simulink model "PTControl"  (Simulink 8.7)
settings: Solver=ode45  StartTime=0.0  StopTime=inf  RelTol=1e-3
libraries: CarMaker4SL x2
(part 3 of 3)

== system PTControl/CarMaker/IPG Vehicle/PowerTrain/PTControl Example/PTControl_In/CreateBus PTC GearBoxM_In3 ==
  In : Inport
  BusCreator : BusCreator  Inputs=20
  Demux : Demux  Outputs=20
  Out : Outport
  wires:
  Demux/20 -> BusCreator/20  "PTC GearBoxM_In3 Clutch_dis i_TrqIn2Out"
  Demux/19 -> BusCreator/19  "PTC GearBoxM_In3 Clutch_dis Trq_out"
  Demux/18 -> BusCreator/18  "PTC GearBoxM_In3 Clutch_dis Trq_in"
  Demux/17 -> BusCreator/17  "PTC GearBoxM_In3 Clutch_dis rotv_out"
  Demux/16 -> BusCreator/16  "PTC GearBoxM_In3 Clutch_dis rotv_in"
  Demux/15 -> BusCreator/15  "PTC GearBoxM_In3 Clutch_dis Pos"
  Demux/14 -> BusCreator/14  "PTC GearBoxM_In3 Clutch i_TrqIn2Out"
  Demux/13 -> BusCreator/13  "PTC GearBoxM_In3 Clutch Trq_out"
  Demux/12 -> BusCreator/12  "PTC GearBoxM_In3 Clutch Trq_in"
  Demux/11 -> BusCreator/11  "PTC GearBoxM_In3 Clutch rotv_out"
  Demux/10 -> BusCreator/10  "PTC GearBoxM_In3 Clutch rotv_in"
  Demux/9 -> BusCreator/9  "PTC GearBoxM_In3 Clutch Pos"
  Demux/8 -> BusCreator/8  "PTC GearBoxM_In3 Trq_out"
  Demux/7 -> BusCreator/7  "PTC GearBoxM_In3 Trq_in"
  Demux/6 -> BusCreator/6  "PTC GearBoxM_In3 rotv_out"
  Demux/5 -> BusCreator/5  "PTC GearBoxM_In3 rotv_in"
  Demux/4 -> BusCreator/4  "PTC GearBoxM_In3 i"
  Demux/3 -> BusCreator/3  "PTC GearBoxM_In3 Trq_DriveSrc_trg"
  Demux/2 -> BusCreator/2  "PTC GearBoxM_In3 GearNo_dis"
  Demux/1 -> BusCreator/1  "PTC GearBoxM_In3 GearNo"
  BusCreator/1 -> Out/1
  In/1 -> Demux/1

== system PTControl/CarMaker/IPG Vehicle/PowerTrain/PTControl Example/PTControl_In/CreateBus PTC ISGIn ==
  In : Inport
  BusCreator : BusCreator  Inputs=9
  Demux : Demux  Outputs=9
  Out : Outport
  wires:
  Demux/9 -> BusCreator/9  "PTC ISGIn i_M2W_RR"
  Demux/8 -> BusCreator/8  "PTC ISGIn i_M2W_RL"
  Demux/7 -> BusCreator/7  "PTC ISGIn i_M2W_FR"
  Demux/6 -> BusCreator/6  "PTC ISGIn i_M2W_FL"
  Demux/5 -> BusCreator/5  "PTC ISGIn PwrElec"
  Demux/4 -> BusCreator/4  "PTC ISGIn TrqGen_max"
  Demux/3 -> BusCreator/3  "PTC ISGIn TrqMot_max"
  Demux/2 -> BusCreator/2  "PTC ISGIn Trq"
  Demux/1 -> BusCreator/1  "PTC ISGIn rotv"
  BusCreator/1 -> Out/1
  In/1 -> Demux/1

== system PTControl/CarMaker/IPG Vehicle/PowerTrain/PTControl Example/PTControl_In/CreateBus PTC MotorIn0 ==
  In : Inport
  BusCreator : BusCreator  Inputs=9
  Demux : Demux  Outputs=9
  Out : Outport
  wires:
  Demux/9 -> BusCreator/9  "PTC MotorIn0 i_M2W_RR"
  Demux/8 -> BusCreator/8  "PTC MotorIn0 i_M2W_RL"
  Demux/7 -> BusCreator/7  "PTC MotorIn0 i_M2W_FR"
  Demux/6 -> BusCreator/6  "PTC MotorIn0 i_M2W_FL"
  Demux/5 -> BusCreator/5  "PTC MotorIn0 PwrElec"
  Demux/4 -> BusCreator/4  "PTC MotorIn0 TrqGen_max"
  Demux/3 -> BusCreator/3  "PTC MotorIn0 TrqMot_max"
  Demux/2 -> BusCreator/2  "PTC MotorIn0 Trq"
  Demux/1 -> BusCreator/1  "PTC MotorIn0 rotv"
  BusCreator/1 -> Out/1
  In/1 -> Demux/1

== system PTControl/CarMaker/IPG Vehicle/PowerTrain/PTControl Example/PTControl_In/CreateBus PTC MotorIn1 ==
  In : Inport
  BusCreator : BusCreator  Inputs=9
  Demux : Demux  Outputs=9
  Out : Outport
  wires:
  Demux/9 -> BusCreator/9  "PTC MotorIn1 i_M2W_RR"
  Demux/8 -> BusCreator/8  "PTC MotorIn1 i_M2W_RL"
  Demux/7 -> BusCreator/7  "PTC MotorIn1 i_M2W_FR"
  Demux/6 -> BusCreator/6  "PTC MotorIn1 i_M2W_FL"
  Demux/5 -> BusCreator/5  "PTC MotorIn1 PwrElec"
  Demux/4 -> BusCreator/4  "PTC MotorIn1 TrqGen_max"
  Demux/3 -> BusCreator/3  "PTC MotorIn1 TrqMot_max"
  Demux/2 -> BusCreator/2  "PTC MotorIn1 Trq"
  Demux/1 -> BusCreator/1  "PTC MotorIn1 rotv"
  BusCreator/1 -> Out/1
  In/1 -> Demux/1

== system PTControl/CarMaker/IPG Vehicle/PowerTrain/PTControl Example/PTControl_In/CreateBus PTC MotorIn2 ==
  In : Inport
  BusCreator : BusCreator  Inputs=9
  Demux : Demux  Outputs=9
  Out : Outport
  wires:
  Demux/9 -> BusCreator/9  "PTC MotorIn2 i_M2W_RR"
  Demux/8 -> BusCreator/8  "PTC MotorIn2 i_M2W_RL"
  Demux/7 -> BusCreator/7  "PTC MotorIn2 i_M2W_FR"
  Demux/6 -> BusCreator/6  "PTC MotorIn2 i_M2W_FL"
  Demux/5 -> BusCreator/5  "PTC MotorIn2 PwrElec"
  Demux/4 -> BusCreator/4  "PTC MotorIn2 TrqGen_max"
  Demux/3 -> BusCreator/3  "PTC MotorIn2 TrqMot_max"
  Demux/2 -> BusCreator/2  "PTC MotorIn2 Trq"
  Demux/1 -> BusCreator/1  "PTC MotorIn2 rotv"
  BusCreator/1 -> Out/1
  In/1 -> Demux/1

== system PTControl/CarMaker/IPG Vehicle/PowerTrain/PTControl Example/PTControl_In/CreateBus PTC MotorIn3 ==
  In : Inport
  BusCreator : BusCreator  Inputs=9
  Demux : Demux  Outputs=9
  Out : Outport
  wires:
  Demux/9 -> BusCreator/9  "PTC MotorIn3 i_M2W_RR"
  Demux/8 -> BusCreator/8  "PTC MotorIn3 i_M2W_RL"
  Demux/7 -> BusCreator/7  "PTC MotorIn3 i_M2W_FR"
  Demux/6 -> BusCreator/6  "PTC MotorIn3 i_M2W_FL"
  Demux/5 -> BusCreator/5  "PTC MotorIn3 PwrElec"
  Demux/4 -> BusCreator/4  "PTC MotorIn3 TrqGen_max"
  Demux/3 -> BusCreator/3  "PTC MotorIn3 TrqMot_max"
  Demux/2 -> BusCreator/2  "PTC MotorIn3 Trq"
  Demux/1 -> BusCreator/1  "PTC MotorIn3 rotv"
  BusCreator/1 -> Out/1
  In/1 -> Demux/1

== system PTControl/CarMaker/IPG Vehicle/PowerTrain/PTControl Example/PTControl_In/CreateBus PTC PwrSupplyIn ==
  In : Inport
  BusCreator : BusCreator  Inputs=12
  Demux : Demux  Outputs=12
  Out : Outport
  wires:
  Demux/12 -> BusCreator/12  "PTC PwrSupplyIn Eta_HV1toHV2"
  Demux/11 -> BusCreator/11  "PTC PwrSupplyIn Eta_HV1toLV"
  Demux/10 -> BusCreator/10  "PTC PwrSupplyIn Pwr_HV1toHV2_max"
  Demux/9 -> BusCreator/9  "PTC PwrSupplyIn Pwr_HV1toLV_max"
  Demux/8 -> BusCreator/8  "PTC PwrSupplyIn Pwr_HV1toHV2"
  Demux/7 -> BusCreator/7  "PTC PwrSupplyIn Pwr_HV1toLV"
  Demux/6 -> BusCreator/6  "PTC PwrSupplyIn Voltage_HV2"
  Demux/5 -> BusCreator/5  "PTC PwrSupplyIn Voltage_HV1"
  Demux/4 -> BusCreator/4  "PTC PwrSupplyIn Voltage_LV"
  Demux/3 -> BusCreator/3  "PTC PwrSupplyIn Pwr_HV2"
  Demux/2 -> BusCreator/2  "PTC PwrSupplyIn Pwr_HV1"
  Demux/1 -> BusCreator/1  "PTC PwrSupplyIn Pwr_LV"
  BusCreator/1 -> Out/1
  In/1 -> Demux/1

== system PTControl/CarMaker/IPG Vehicle/PowerTrain/PTControl Example/PTControl_In/CreateBus PTC Vehicle Ctrl ==
  In : Inport
  BusCreator : BusCreator  Inputs=8
  Demux : Demux  Outputs=8
  Out : Outport
  wires:
  Demux/8 -> BusCreator/8  "PTC Velocity"
  Demux/7 -> BusCreator/7  "PTC Brake"
  Demux/6 -> BusCreator/6  "PTC Gas"
  Demux/5 -> BusCreator/5  "PTC Clutch"
  Demux/4 -> BusCreator/4  "PTC GearNoTrg"
  Demux/3 -> BusCreator/3  "PTC SelectorCtrl"
  Demux/2 -> BusCreator/2  "PTC SST"
  Demux/1 -> BusCreator/1  "PTC Key"
  BusCreator/1 -> Out/1
  In/1 -> Demux/1

== system PTControl/CarMaker/IPG Vehicle/PowerTrain/PTControl Example/PTControl_In/CreateBus PTC WheelIn ==
  In : Inport
  BusCreator : BusCreator  Inputs=4
  Demux : Demux
  Out : Outport
  wires:
  Demux/4 -> BusCreator/4  "PTC WheelIn_RR Trq_BrakeReg_trg"
  Demux/3 -> BusCreator/3  "PTC WheelIn_RL Trq_BrakeReg_trg"
  Demux/2 -> BusCreator/2  "PTC WheelIn_FR Trq_BrakeReg_trg"
  Demux/1 -> BusCreator/1  "PTC WheelIn_FL Trq_BrakeReg_trg"
  BusCreator/1 -> Out/1
  In/1 -> Demux/1

== system PTControl/CarMaker/IPG Vehicle/PowerTrain/PTControl Example/PTControl_In/CreateBus PTC_Cfg Battery ==
  In : Inport
  BusCreator : BusCreator  Inputs=8
  Demux : Demux  Outputs=8
  Out : Outport
  wires:
  Demux/8 -> BusCreator/8  "PTC_Cfg BattHV Voltage"
  Demux/7 -> BusCreator/7  "PTC_Cfg BattHV Capacity"
  Demux/6 -> BusCreator/6  "PTC_Cfg BattHV SOC_max"
  Demux/5 -> BusCreator/5  "PTC_Cfg BattHV SOC_min"
  Demux/4 -> BusCreator/4  "PTC_Cfg BattLV Voltage"
  Demux/3 -> BusCreator/3  "PTC_Cfg BattLV Capacity"
  Demux/2 -> BusCreator/2  "PTC_Cfg BattLV SOC_max"
  Demux/1 -> BusCreator/1  "PTC_Cfg BattLV SOC_min"
  BusCreator/1 -> Out/1
  In/1 -> Demux/1

== system PTControl/CarMaker/IPG Vehicle/PowerTrain/PTControl Example/PTControl_In/CreateBus PTC_Cfg Engine ==
  In : Inport
  BusCreator : BusCreator  Inputs=4
  Demux : Demux
  Out : Outport
  wires:
  Demux/4 -> BusCreator/4  "PTC_Cfg Engine rotv_opt"
  Demux/3 -> BusCreator/3  "PTC_Cfg Engine rotv_idle"
  Demux/2 -> BusCreator/2  "PTC_Cfg Engine rotv_max"
  Demux/1 -> BusCreator/1  "PTC_Cfg Engine Fuel_l2kWh"
  BusCreator/1 -> Out/1
  In/1 -> Demux/1

== system PTControl/CarMaker/IPG Vehicle/PowerTrain/PTControl Example/PTControl_In/CreateBus PTC_Cfg GearBox ==
  In : Inport
  BusCreator : BusCreator  Inputs=38
  Demux : Demux  Outputs=38
  Out : Outport
  wires:
  Demux/38 -> BusCreator/38  "PTC_Cfg GearBox iBGear16"
  Demux/37 -> BusCreator/37  "PTC_Cfg GearBox iBGear15"
  Demux/36 -> BusCreator/36  "PTC_Cfg GearBox iBGear14"
  Demux/35 -> BusCreator/35  "PTC_Cfg GearBox iBGear13"
  Demux/34 -> BusCreator/34  "PTC_Cfg GearBox iBGear12"
  Demux/33 -> BusCreator/33  "PTC_Cfg GearBox iBGear11"
  Demux/32 -> BusCreator/32  "PTC_Cfg GearBox iBGear10"
  Demux/31 -> BusCreator/31  "PTC_Cfg GearBox iBGear9"
  Demux/30 -> BusCreator/30  "PTC_Cfg GearBox iBGear8"
  Demux/29 -> BusCreator/29  "PTC_Cfg GearBox iBGear7"
  Demux/28 -> BusCreator/28  "PTC_Cfg GearBox iBGear6"
  Demux/27 -> BusCreator/27  "PTC_Cfg GearBox iBGear5"
  Demux/26 -> BusCreator/26  "PTC_Cfg GearBox iBGear4"
  Demux/25 -> BusCreator/25  "PTC_Cfg GearBox iBGear3"
  Demux/24 -> BusCreator/24  "PTC_Cfg GearBox iBGear2"
  Demux/23 -> BusCreator/23  "PTC_Cfg GearBox iBGear1"
  Demux/22 -> BusCreator/22  "PTC_Cfg GearBox iBGear0"
  Demux/21 -> BusCreator/21  "PTC_Cfg GearBox nBGears"
  Demux/20 -> BusCreator/20  "PTC_Cfg GearBox iFGear16"
  Demux/19 -> BusCreator/19  "PTC_Cfg GearBox iFGear15"
  Demux/18 -> BusCreator/18  "PTC_Cfg GearBox iFGear14"
  Demux/17 -> BusCreator/17  "PTC_Cfg GearBox iFGear13"
  Demux/16 -> BusCreator/16  "PTC_Cfg GearBox iFGear12"
  Demux/15 -> BusCreator/15  "PTC_Cfg GearBox iFGear11"
  Demux/14 -> BusCreator/14  "PTC_Cfg GearBox iFGear10"
  Demux/13 -> BusCreator/13  "PTC_Cfg GearBox iFGear9"
  Demux/12 -> BusCreator/12  "PTC_Cfg GearBox iFGear8"
  Demux/11 -> BusCreator/11  "PTC_Cfg GearBox iFGear7"
  Demux/10 -> BusCreator/10  "PTC_Cfg GearBox iFGear6"
  Demux/9 -> BusCreator/9  "PTC_Cfg GearBox iFGear5"
  Demux/8 -> BusCreator/8  "PTC_Cfg GearBox iFGear4"
  Demux/7 -> BusCreator/7  "PTC_Cfg GearBox iFGear3"
  Demux/6 -> BusCreator/6  "PTC_Cfg GearBox iFGear2"
  Demux/5 -> BusCreator/5  "PTC_Cfg GearBox iFGear1"
  Demux/4 -> BusCreator/4  "PTC_Cfg GearBox iFGear0"
  Demux/3 -> BusCreator/3  "PTC_Cfg GearBox nFGears"
  Demux/2 -> BusCreator/2  "PTC_Cfg GearBox ClKind"
  Demux/1 -> BusCreator/1  "PTC_Cfg GearBox GBKind"
  BusCreator/1 -> Out/1
  In/1 -> Demux/1

== system PTControl/CarMaker/IPG Vehicle/PowerTrain/PTControl Example/PTControl_In/CreateBus PTC_Cfg GearBoxM0 ==
  In : Inport
  BusCreator : BusCreator  Inputs=38
  Demux : Demux  Outputs=38
  Out : Outport
  wires:
  Demux/38 -> BusCreator/38  "PTC_Cfg GearBoxM0 iBGear16"
  Demux/37 -> BusCreator/37  "PTC_Cfg GearBoxM0 iBGear15"
  Demux/36 -> BusCreator/36  "PTC_Cfg GearBoxM0 iBGear14"
  Demux/35 -> BusCreator/35  "PTC_Cfg GearBoxM0 iBGear13"
  Demux/34 -> BusCreator/34  "PTC_Cfg GearBoxM0 iBGear12"
  Demux/33 -> BusCreator/33  "PTC_Cfg GearBoxM0 iBGear11"
  Demux/32 -> BusCreator/32  "PTC_Cfg GearBoxM0 iBGear10"
  Demux/31 -> BusCreator/31  "PTC_Cfg GearBoxM0 iBGear9"
  Demux/30 -> BusCreator/30  "PTC_Cfg GearBoxM0 iBGear8"
  Demux/29 -> BusCreator/29  "PTC_Cfg GearBoxM0 iBGear7"
  Demux/28 -> BusCreator/28  "PTC_Cfg GearBoxM0 iBGear6"
  Demux/27 -> BusCreator/27  "PTC_Cfg GearBoxM0 iBGear5"
  Demux/26 -> BusCreator/26  "PTC_Cfg GearBoxM0 iBGear4"
  Demux/25 -> BusCreator/25  "PTC_Cfg GearBoxM0 iBGear3"
  Demux/24 -> BusCreator/24  "PTC_Cfg GearBoxM0 iBGear2"
  Demux/23 -> BusCreator/23  "PTC_Cfg GearBoxM0 iBGear1"
  Demux/22 -> BusCreator/22  "PTC_Cfg GearBoxM0 iBGear0"
  Demux/21 -> BusCreator/21  "PTC_Cfg GearBoxM0 nBGears"
  Demux/20 -> BusCreator/20  "PTC_Cfg GearBoxM0 iFGear16"
  Demux/19 -> BusCreator/19  "PTC_Cfg GearBoxM0 iFGear15"
  Demux/18 -> BusCreator/18  "PTC_Cfg GearBoxM0 iFGear14"
  Demux/17 -> BusCreator/17  "PTC_Cfg GearBoxM0 iFGear13"
  Demux/16 -> BusCreator/16  "PTC_Cfg GearBoxM0 iFGear12"
  Demux/15 -> BusCreator/15  "PTC_Cfg GearBoxM0 iFGear11"
  Demux/14 -> BusCreator/14  "PTC_Cfg GearBoxM0 iFGear10"
  Demux/13 -> BusCreator/13  "PTC_Cfg GearBoxM0 iFGear9"
  Demux/12 -> BusCreator/12  "PTC_Cfg GearBoxM0 iFGear8"
  Demux/11 -> BusCreator/11  "PTC_Cfg GearBoxM0 iFGear7"
  Demux/10 -> BusCreator/10  "PTC_Cfg GearBoxM0 iFGear6"
  Demux/9 -> BusCreator/9  "PTC_Cfg GearBoxM0 iFGear5"
  Demux/8 -> BusCreator/8  "PTC_Cfg GearBoxM0 iFGear4"
  Demux/7 -> BusCreator/7  "PTC_Cfg GearBoxM0 iFGear3"
  Demux/6 -> BusCreator/6  "PTC_Cfg GearBoxM0 iFGear2"
  Demux/5 -> BusCreator/5  "PTC_Cfg GearBoxM0 iFGear1"
  Demux/4 -> BusCreator/4  "PTC_Cfg GearBoxM0 iFGear0"
  Demux/3 -> BusCreator/3  "PTC_Cfg GearBoxM0 nFGears"
  Demux/2 -> BusCreator/2  "PTC_Cfg GearBoxM0 ClKind"
  Demux/1 -> BusCreator/1  "PTC_Cfg GearBoxM0 GBKind"
  BusCreator/1 -> Out/1
  In/1 -> Demux/1

== system PTControl/CarMaker/IPG Vehicle/PowerTrain/PTControl Example/PTControl_In/CreateBus PTC_Cfg GearBoxM1 ==
  In : Inport
  BusCreator : BusCreator  Inputs=38
  Demux : Demux  Outputs=38
  Out : Outport
  wires:
  Demux/38 -> BusCreator/38  "PTC_Cfg GearBoxM1 iBGear16"
  Demux/37 -> BusCreator/37  "PTC_Cfg GearBoxM1 iBGear15"
  Demux/36 -> BusCreator/36  "PTC_Cfg GearBoxM1 iBGear14"
  Demux/35 -> BusCreator/35  "PTC_Cfg GearBoxM1 iBGear13"
  Demux/34 -> BusCreator/34  "PTC_Cfg GearBoxM1 iBGear12"
  Demux/33 -> BusCreator/33  "PTC_Cfg GearBoxM1 iBGear11"
  Demux/32 -> BusCreator/32  "PTC_Cfg GearBoxM1 iBGear10"
  Demux/31 -> BusCreator/31  "PTC_Cfg GearBoxM1 iBGear9"
  Demux/30 -> BusCreator/30  "PTC_Cfg GearBoxM1 iBGear8"
  Demux/29 -> BusCreator/29  "PTC_Cfg GearBoxM1 iBGear7"
  Demux/28 -> BusCreator/28  "PTC_Cfg GearBoxM1 iBGear6"
  Demux/27 -> BusCreator/27  "PTC_Cfg GearBoxM1 iBGear5"
  Demux/26 -> BusCreator/26  "PTC_Cfg GearBoxM1 iBGear4"
  Demux/25 -> BusCreator/25  "PTC_Cfg GearBoxM1 iBGear3"
  Demux/24 -> BusCreator/24  "PTC_Cfg GearBoxM1 iBGear2"
  Demux/23 -> BusCreator/23  "PTC_Cfg GearBoxM1 iBGear1"
  Demux/22 -> BusCreator/22  "PTC_Cfg GearBoxM1 iBGear0"
  Demux/21 -> BusCreator/21  "PTC_Cfg GearBoxM1 nBGears"
  Demux/20 -> BusCreator/20  "PTC_Cfg GearBoxM1 iFGear16"
  Demux/19 -> BusCreator/19  "PTC_Cfg GearBoxM1 iFGear15"
  Demux/18 -> BusCreator/18  "PTC_Cfg GearBoxM1 iFGear14"
  Demux/17 -> BusCreator/17  "PTC_Cfg GearBoxM1 iFGear13"
  Demux/16 -> BusCreator/16  "PTC_Cfg GearBoxM1 iFGear12"
  Demux/15 -> BusCreator/15  "PTC_Cfg GearBoxM1 iFGear11"
  Demux/14 -> BusCreator/14  "PTC_Cfg GearBoxM1 iFGear10"
  Demux/13 -> BusCreator/13  "PTC_Cfg GearBoxM1 iFGear9"
  Demux/12 -> BusCreator/12  "PTC_Cfg GearBoxM1 iFGear8"
  Demux/11 -> BusCreator/11  "PTC_Cfg GearBoxM1 iFGear7"
  Demux/10 -> BusCreator/10  "PTC_Cfg GearBoxM1 iFGear6"
  Demux/9 -> BusCreator/9  "PTC_Cfg GearBoxM1 iFGear5"
  Demux/8 -> BusCreator/8  "PTC_Cfg GearBoxM1 iFGear4"
  Demux/7 -> BusCreator/7  "PTC_Cfg GearBoxM1 iFGear3"
  Demux/6 -> BusCreator/6  "PTC_Cfg GearBoxM1 iFGear2"
  Demux/5 -> BusCreator/5  "PTC_Cfg GearBoxM1 iFGear1"
  Demux/4 -> BusCreator/4  "PTC_Cfg GearBoxM1 iFGear0"
  Demux/3 -> BusCreator/3  "PTC_Cfg GearBoxM1 nFGears"
  Demux/2 -> BusCreator/2  "PTC_Cfg GearBoxM1 ClKind"
  Demux/1 -> BusCreator/1  "PTC_Cfg GearBoxM1 GBKind"
  BusCreator/1 -> Out/1
  In/1 -> Demux/1

== system PTControl/CarMaker/IPG Vehicle/PowerTrain/PTControl Example/PTControl_In/CreateBus PTC_Cfg GearBoxM2 ==
  In : Inport
  BusCreator : BusCreator  Inputs=38
  Demux : Demux  Outputs=38
  Out : Outport
  wires:
  Demux/38 -> BusCreator/38  "PTC_Cfg GearBoxM2 iBGear16"
  Demux/37 -> BusCreator/37  "PTC_Cfg GearBoxM2 iBGear15"
  Demux/36 -> BusCreator/36  "PTC_Cfg GearBoxM2 iBGear14"
  Demux/35 -> BusCreator/35  "PTC_Cfg GearBoxM2 iBGear13"
  Demux/34 -> BusCreator/34  "PTC_Cfg GearBoxM2 iBGear12"
  Demux/33 -> BusCreator/33  "PTC_Cfg GearBoxM2 iBGear11"
  Demux/32 -> BusCreator/32  "PTC_Cfg GearBoxM2 iBGear10"
  Demux/31 -> BusCreator/31  "PTC_Cfg GearBoxM2 iBGear9"
  Demux/30 -> BusCreator/30  "PTC_Cfg GearBoxM2 iBGear8"
  Demux/29 -> BusCreator/29  "PTC_Cfg GearBoxM2 iBGear7"
  Demux/28 -> BusCreator/28  "PTC_Cfg GearBoxM2 iBGear6"
  Demux/27 -> BusCreator/27  "PTC_Cfg GearBoxM2 iBGear5"
  Demux/26 -> BusCreator/26  "PTC_Cfg GearBoxM2 iBGear4"
  Demux/25 -> BusCreator/25  "PTC_Cfg GearBoxM2 iBGear3"
  Demux/24 -> BusCreator/24  "PTC_Cfg GearBoxM2 iBGear2"
  Demux/23 -> BusCreator/23  "PTC_Cfg GearBoxM2 iBGear1"
  Demux/22 -> BusCreator/22  "PTC_Cfg GearBoxM2 iBGear0"
  Demux/21 -> BusCreator/21  "PTC_Cfg GearBoxM2 nBGears"
  Demux/20 -> BusCreator/20  "PTC_Cfg GearBoxM2 iFGear16"
  Demux/19 -> BusCreator/19  "PTC_Cfg GearBoxM2 iFGear15"
  Demux/18 -> BusCreator/18  "PTC_Cfg GearBoxM2 iFGear14"
  Demux/17 -> BusCreator/17  "PTC_Cfg GearBoxM2 iFGear13"
  Demux/16 -> BusCreator/16  "PTC_Cfg GearBoxM2 iFGear12"
  Demux/15 -> BusCreator/15  "PTC_Cfg GearBoxM2 iFGear11"
  Demux/14 -> BusCreator/14  "PTC_Cfg GearBoxM2 iFGear10"
  Demux/13 -> BusCreator/13  "PTC_Cfg GearBoxM2 iFGear9"
  Demux/12 -> BusCreator/12  "PTC_Cfg GearBoxM2 iFGear8"
  Demux/11 -> BusCreator/11  "PTC_Cfg GearBoxM2 iFGear7"
  Demux/10 -> BusCreator/10  "PTC_Cfg GearBoxM2 iFGear6"
  Demux/9 -> BusCreator/9  "PTC_Cfg GearBoxM2 iFGear5"
  Demux/8 -> BusCreator/8  "PTC_Cfg GearBoxM2 iFGear4"
  Demux/7 -> BusCreator/7  "PTC_Cfg GearBoxM2 iFGear3"
  Demux/6 -> BusCreator/6  "PTC_Cfg GearBoxM2 iFGear2"
  Demux/5 -> BusCreator/5  "PTC_Cfg GearBoxM2 iFGear1"
  Demux/4 -> BusCreator/4  "PTC_Cfg GearBoxM2 iFGear0"
  Demux/3 -> BusCreator/3  "PTC_Cfg GearBoxM2 nFGears"
  Demux/2 -> BusCreator/2  "PTC_Cfg GearBoxM2 ClKind"
  Demux/1 -> BusCreator/1  "PTC_Cfg GearBoxM2 GBKind"
  BusCreator/1 -> Out/1
  In/1 -> Demux/1

== system PTControl/CarMaker/IPG Vehicle/PowerTrain/PTControl Example/PTControl_In/CreateBus PTC_Cfg GearBoxM3 ==
  In : Inport
  BusCreator : BusCreator  Inputs=38
  Demux : Demux  Outputs=38
  Out : Outport
  wires:
  Demux/38 -> BusCreator/38  "PTC_Cfg GearBoxM3 iBGear16"
  Demux/37 -> BusCreator/37  "PTC_Cfg GearBoxM3 iBGear15"
  Demux/36 -> BusCreator/36  "PTC_Cfg GearBoxM3 iBGear14"
  Demux/35 -> BusCreator/35  "PTC_Cfg GearBoxM3 iBGear13"
  Demux/34 -> BusCreator/34  "PTC_Cfg GearBoxM3 iBGear12"
  Demux/33 -> BusCreator/33  "PTC_Cfg GearBoxM3 iBGear11"
  Demux/32 -> BusCreator/32  "PTC_Cfg GearBoxM3 iBGear10"
  Demux/31 -> BusCreator/31  "PTC_Cfg GearBoxM3 iBGear9"
  Demux/30 -> BusCreator/30  "PTC_Cfg GearBoxM3 iBGear8"
  Demux/29 -> BusCreator/29  "PTC_Cfg GearBoxM3 iBGear7"
  Demux/28 -> BusCreator/28  "PTC_Cfg GearBoxM3 iBGear6"
  Demux/27 -> BusCreator/27  "PTC_Cfg GearBoxM3 iBGear5"
  Demux/26 -> BusCreator/26  "PTC_Cfg GearBoxM3 iBGear4"
  Demux/25 -> BusCreator/25  "PTC_Cfg GearBoxM3 iBGear3"
  Demux/24 -> BusCreator/24  "PTC_Cfg GearBoxM3 iBGear2"
  Demux/23 -> BusCreator/23  "PTC_Cfg GearBoxM3 iBGear1"
  Demux/22 -> BusCreator/22  "PTC_Cfg GearBoxM3 iBGear0"
  Demux/21 -> BusCreator/21  "PTC_Cfg GearBoxM3 nBGears"
  Demux/20 -> BusCreator/20  "PTC_Cfg GearBoxM3 iFGear16"
  Demux/19 -> BusCreator/19  "PTC_Cfg GearBoxM3 iFGear15"
  Demux/18 -> BusCreator/18  "PTC_Cfg GearBoxM3 iFGear14"
  Demux/17 -> BusCreator/17  "PTC_Cfg GearBoxM3 iFGear13"
  Demux/16 -> BusCreator/16  "PTC_Cfg GearBoxM3 iFGear12"
  Demux/15 -> BusCreator/15  "PTC_Cfg GearBoxM3 iFGear11"
  Demux/14 -> BusCreator/14  "PTC_Cfg GearBoxM3 iFGear10"
  Demux/13 -> BusCreator/13  "PTC_Cfg GearBoxM3 iFGear9"
  Demux/12 -> BusCreator/12  "PTC_Cfg GearBoxM3 iFGear8"
  Demux/11 -> BusCreator/11  "PTC_Cfg GearBoxM3 iFGear7"
  Demux/10 -> BusCreator/10  "PTC_Cfg GearBoxM3 iFGear6"
  Demux/9 -> BusCreator/9  "PTC_Cfg GearBoxM3 iFGear5"
  Demux/8 -> BusCreator/8  "PTC_Cfg GearBoxM3 iFGear4"
  Demux/7 -> BusCreator/7  "PTC_Cfg GearBoxM3 iFGear3"
  Demux/6 -> BusCreator/6  "PTC_Cfg GearBoxM3 iFGear2"
  Demux/5 -> BusCreator/5  "PTC_Cfg GearBoxM3 iFGear1"
  Demux/4 -> BusCreator/4  "PTC_Cfg GearBoxM3 iFGear0"
  Demux/3 -> BusCreator/3  "PTC_Cfg GearBoxM3 nFGears"
  Demux/2 -> BusCreator/2  "PTC_Cfg GearBoxM3 ClKind"
  Demux/1 -> BusCreator/1  "PTC_Cfg GearBoxM3 GBKind"
  BusCreator/1 -> Out/1
  In/1 -> Demux/1

== system PTControl/CarMaker/IPG Vehicle/PowerTrain/PTControl Example/PTControl_In/CreateBus PTC_Cfg ISG ==
  In : Inport
  BusCreator : BusCreator  Inputs=4
  Demux : Demux
  Out : Outport
  wires:
  Demux/4 -> BusCreator/4  "PTC_Cfg ISG rotv_Gen_max"
  Demux/3 -> BusCreator/3  "PTC_Cfg ISG rotv_Mot_max"
  Demux/2 -> BusCreator/2  "PTC_Cfg ISG Ratio"
  Demux/1 -> BusCreator/1  "PTC_Cfg ISG Level"
  BusCreator/1 -> Out/1
  In/1 -> Demux/1

== system PTControl/CarMaker/IPG Vehicle/PowerTrain/PTControl Example/PTControl_In/CreateBus PTC_Cfg Misc ==
  In : Inport
  BusCreator : BusCreator  Inputs=13
  Demux : Demux  Outputs=13
  Out : Outport
  wires:
  Demux/13 -> BusCreator/13  "PTC_Cfg DriveSourcePos3"
  Demux/12 -> BusCreator/12  "PTC_Cfg DriveSourcePos2"
  Demux/11 -> BusCreator/11  "PTC_Cfg DriveSourcePos1"
  Demux/10 -> BusCreator/10  "PTC_Cfg DriveSourcePos0"
  Demux/9 -> BusCreator/9  "PTC_Cfg DL_iDiff_mean"
  Demux/8 -> BusCreator/8  "PTC_Cfg Aero_Frcx"
  Demux/7 -> BusCreator/7  "PTC_Cfg WheelRadius"
  Demux/6 -> BusCreator/6  "PTC_Cfg Vehicle_nWheels"
  Demux/5 -> BusCreator/5  "PTC_Cfg nPlanetGear"
  Demux/4 -> BusCreator/4  "PTC_Cfg nGearBoxM"
  Demux/3 -> BusCreator/3  "PTC_Cfg nMotor"
  Demux/2 -> BusCreator/2  "PTC_Cfg ClKind"
  Demux/1 -> BusCreator/1  "PTC_Cfg PTKind"
  BusCreator/1 -> Out/1
  In/1 -> Demux/1

== system PTControl/CarMaker/IPG Vehicle/PowerTrain/PTControl Example/PTControl_In/CreateBus PTC_Cfg Motor ==
  In : Inport
  BusCreator : BusCreator  Inputs=16
  Demux : Demux  Outputs=16
  Out : Outport
  wires:
  Demux/16 -> BusCreator/16  "PTC_Cfg Motor3 rotv_Gen_max"
  Demux/15 -> BusCreator/15  "PTC_Cfg Motor3 rotv_Mot_max"
  Demux/14 -> BusCreator/14  "PTC_Cfg Motor3 Ratio"
  Demux/13 -> BusCreator/13  "PTC_Cfg Motor3 Level"
  Demux/12 -> BusCreator/12  "PTC_Cfg Motor2 rotv_Gen_max"
  Demux/11 -> BusCreator/11  "PTC_Cfg Motor2 rotv_Mot_max"
  Demux/10 -> BusCreator/10  "PTC_Cfg Motor2 Ratio"
  Demux/9 -> BusCreator/9  "PTC_Cfg Motor2 Level"
  Demux/8 -> BusCreator/8  "PTC_Cfg Motor1 rotv_Gen_max"
  Demux/7 -> BusCreator/7  "PTC_Cfg Motor1 rotv_Mot_max"
  Demux/6 -> BusCreator/6  "PTC_Cfg Motor1 Ratio"
  Demux/5 -> BusCreator/5  "PTC_Cfg Motor1 Level"
  Demux/4 -> BusCreator/4  "PTC_Cfg Motor0 rotv_Gen_max"
  Demux/3 -> BusCreator/3  "PTC_Cfg Motor0 rotv_Mot_max"
  Demux/2 -> BusCreator/2  "PTC_Cfg Motor0 Ratio"
  Demux/1 -> BusCreator/1  "PTC_Cfg Motor0 Level"
  BusCreator/1 -> Out/1
  In/1 -> Demux/1

== system PTControl/CarMaker/IPG Vehicle/PowerTrain/PTControl Example/PTControl_In/CreateBus PTC_Cfg PlanetGear ==
  In : Inport
  BusCreator : BusCreator  Inputs=1
  Demux : Demux  Outputs=1
  Out : Outport
  wires:
  Demux/1 -> BusCreator/1  "PTC_Cfg PlanetGear0 Ratio"
  BusCreator/1 -> Out/1
  In/1 -> Demux/1
